simulink model "WaveStar"  (R2021b)
settings: Solver=ode4  StartTime=0  StopTime=200  FixedStep=0.01  MaxStep=0.01  RelTol=1e-3  EnableMultiTasking=on
values from neighbouring files (symbols this model uses):
  Ad = sysD.A    [controller_init.m]
  alpha_efft = 1000    [controller_init.m]
  Bd = sysD.B    [controller_init.m]
  cc = 16.70    (= 16.7)    [controller_init.m]
  dt = 10/1000    (= 0.01)    [controller_init.m]    (also in state_space_model_simulation.m = mean(diff(output.wave.time)); transformation_Forces_to_Moments.m = mean(diff(timePlot)))
  eta_generator = 0.7    [controller_init.m]
  eta_motoring = 1 / 0.7    (= 1.42857142857)    [controller_init.m]
  L_AB = 0.412    [Model_Parameters.m]    (also in controller_init.m)
  L_AC = 0.2    [Model_Parameters.m]    (also in controller_init.m)
  LAfloat = 0.54875    [controller_init.m]
  McSat = 12    [controller_init.m]
  Np = 100    [controller_init.m]
  offset_eff = ( eta_motoring + eta_generator ) / 2    (= 1.06428571429)    [controller_init.m]
  Qkf = blkdiag( Qp, Qv, QradM, QexcM )    [controller_init.m]
  qnl = [ 0, 1 ... (first row only)    [controller_init.m]
  R_ctrl = r_ctrl*eye( Np*nu )    [controller_init.m]
  Rkf = blkdiag( Rp, Rv )    [controller_init.m]
  scaler_eff = 1*( eta_motoring - eta_generator ) / 2    (= 0.364285714286)    [controller_init.m]
  simu = simulationClass()    [wecSimInputFile.m]
  Theta0 = deg2rad(26.9527)    [controller_init.m]
  Umax = 12    [controller_init.m]
  Umin = -Umax    (= -12)    [controller_init.m]
  waves = waveClass('etaImport')    [wecSimInputFile.m]
  xPcTs = dt    (= 0.01)    [controller_init.m]
undefined symbols (not defined in the file or in its folder): body, constraint, HPfreq, hydroData, LPfreq, pto, X, Y, Z
libraries: nesl_utility x31, sm_lib x21, WECSim_Lib_Body_Elements x10, WECSim_Lib_Constraints x5, vrlib x1, WECSim_Lib_Frames x1
(part 4 of 4)

== matlab function WaveStar/NMPC - Controller/RTI - NMPC - Algorithm/Compute extracted Energy//Power ==
  data: vel input; P output; tor input; E output; eta_generator parameter; eta_motoring parameter; dt parameter
function [P, E] = extrPower(vel,tor, eta_generator, eta_motoring, dt)
                % Initial conditions
                persistent extractedEnergy 
                if isempty(extractedEnergy)
                    extractedEnergy = 0;
                end

               if vel*tor < 0
                    effi_nmpc = eta_generator;
                else
                    effi_nmpc = eta_motoring;
                end

                extractedPower  = - effi_nmpc*vel*tor;
                extractedEnergy = extractedEnergy + dt*extractedPower;          %Energy absorbed

        P = extractedPower;
        E = extractedEnergy;

== matlab function WaveStar/Float/Hydrodynamic Body/Yaw Kinematic Transforms/With B2B/Yaw Kinematic Transforms ==
  data: yawNonLin input; dispLoc output; dispGlobal input; velGlobal input; accGlobal input; velLoc output; accLoc output; numBody parameter
function [dispLoc, velLoc, accLoc] = kinYawTransformB2B(yawNonLin, dispGlobal, velGlobal, accGlobal, numBody)

[dispLoc, velLoc, accLoc] = kinYawTransformB2B(yawNonLin, dispGlobal, velGlobal, accGlobal, numBody);

end

== matlab function WaveStar/Float/Hydrodynamic Body/Morison Element and Viscous Damping Force Calculation/Morison Element Variant Subsystem/Morison Element On/Regular Wave Morison Force/MATLAB Function ==
  data: z input; f output; r input; Vel input; Accel input; Disp input; Area input; Cd input; Vol input; Ca input; Time input; rho input; waveDir input; waterDepth input; k input; w input; A input; rampTime input; g input; currentSpeed input; currentDirection input; currentDepth input; currentOption input; simuMorison input
function f = regWaveMorison(z,r,Vel,Accel,Disp,Area,Cd,Vol,Ca,Time,rho,waveDir,waterDepth,k,w,A,rampTime,g,currentSpeed,currentDirection,currentDepth,currentOption,simuMorison)

f = regWaveMorison(z,r,Vel,Accel,Disp,Area,Cd,Vol,Ca,Time,rho,waveDir,waterDepth,k,w,A,rampTime,g,currentSpeed,currentDirection,currentDepth,currentOption,simuMorison);

end

== matlab function WaveStar/NMPC - Controller/lin2rot conversion/Linear2Angular Conversion/MATLAB Function1 K [m] ==
  data: u input; y output; L_AB parameter; L_AC parameter
function y = fcn(u,L_AB,L_AC)
%#codegen
y = L_AB'*L_AC'*sin(u);

== matlab function WaveStar/NMPC - Controller/lin2rot conversion/Linear2Angular Conversion/MATLAB Function1 L_BC [m] ==
  data: u input; y output; L_BC_neutral parameter
 function y = fcn(u,L_BC_neutral)
%#codegen
%
y = u+L_BC_neutral';

== matlab function WaveStar/NMPC - Controller/lin2rot conversion/Linear2Angular Conversion/MATLAB Function1 Theta [rad] ==
  data: u input; y output; a_CAB_neutral parameter
function y = fcn(u,a_CAB_neutral)
%#codegen
y = u-a_CAB_neutral';

== matlab function WaveStar/NMPC - Controller/Transform excitation forces in excitation Moment around A ==
  data: theta input; u input; y output; LAfloat parameter; Theta0 parameter
function y = fcn(theta, u, LAfloat, Theta0)

xFexc = u( 1 );
zFexc = u( 3 );
pitchMexc = u( 5 );

y = (-LAfloat * xFexc .*sin( Theta0 + theta ) - zFexc * LAfloat.*cos( Theta0 + theta ) + pitchMexc );

== matlab function WaveStar/NMPC - Controller/lin2rot conversion/Linear2Angular Conversion/MATLAB Function1 a_CAB [rad] ==
  data: u input; y output; L_AB parameter; L_AC parameter
function y = fcn(u,L_AB,L_AC)
%#codegen
%
y = acos((u.^2-L_AB'^2-L_AC'^2)/(-2*L_AB'*L_AC'));

== matlab function WaveStar/Float/Hydrodynamic Body/Hydrostatic Restoring Force Calculation/Linear and Nonlinear Restoring Force Variant Subsystem/Nonlinear Hydrostatic Restoring Force/Restoring Forces ==
  data: x input; elv input; center input; f output; tnorm input; area input; rho input; g input; cg input; p output; mass input
function [f,p]  = nonLinearBuoyancy(x,elv,center,tnorm,area,rho,g,cg,mass)

[f,p]  = nonLinearBuoyancy(x,elv,center,tnorm,area,rho,g,cg,mass);

end
